simulink model "LCK_old"  (R2018b)
settings: Solver=FixedStepDiscrete  StartTime=0.0  StopTime=inf  FixedStep=0.005  RelTol=1e-3
PostLoadFcn:
  | if any(exist('dsrtsu_mdlpostloadfcn', 'file') ~= 0), dsrtsu_mdlpostloadfcn('Execute', bdroot); end
values from neighbouring files (symbols this model uses):
  C_DEG2RAD = 0.0175    [LCK_Macro.sldd]
  C_KPH2MPS = 0.2778    [LCK_Macro.sldd]
  C_NEARZERO = 0.0001    [LCK_Macro.sldd]
  C_ONE = 1.0    [LCK_Macro.sldd]
  C_RAD2DEG = 57.2958    [LCK_Macro.sldd]
  C_ZERO = 0.0    [LCK_Macro.sldd]
  k_accel_pedal_pos_per_speed_x : value not decoded    [LCK_LogicPara.sldd]
  k_accel_pedal_pos_per_speed_z : value not decoded    [LCK_LogicPara.sldd]
  k_brake_suprress_hold = 1000.0    [LCK_LogicPara.sldd]
  k_driver_appl_torque_filt = 50.0    [LCK_LogicPara.sldd]
  k_driver_suppression_hold_time = 3000.0    [LCK_LogicPara.sldd]
  k_hands_on_wheel_hold_msec = 500.0    [LCK_LogicPara.sldd]
  k_hands_on_wheel_torque_hi = 0.2    [LCK_LogicPara.sldd]
  k_hands_on_wheel_torque_lo = 0.15    [LCK_LogicPara.sldd]
  k_handsoff_delay_cycles = 50.0    [LCK_LogicPara.sldd]
  k_handsoff_torq_Lo_CR = 0.3    [LCK_LogicPara.sldd]
  k_handson_delay_cycles = 5.0    [LCK_LogicPara.sldd]
  k_HighAccel_suppress_hold = 3000.0    [LCK_LogicPara.sldd]
  k_HLR_suprress_hold = 3000.0    [LCK_LogicPara.sldd]
  k_hs_StrAng_CR_threshold_z : value not decoded    [LCK_LogicPara.sldd]
  k_LC_Exit_Switch = 0.0    [LCK_LogicPara.sldd]
  k_LCG_Configured = 1.0    [LCK_LogicPara.sldd]
  k_LCK_A0_Rdy2Act_UseConst = 0.0    [LCK_LogicPara.sldd]
  k_LCK_A0Fac_ActSta : value not decoded    [LCK_CtrlPara.sldd]
  k_LCK_A0Fac_DrvStm : value not decoded    [LCK_CtrlPara.sldd]
  k_LCK_A0Shift_LftCurv : value not decoded    [LCK_CtrlPara.sldd]
  k_LCK_A0Shift_RgtCurv : value not decoded    [LCK_CtrlPara.sldd]
  k_LCK_A0Shift_StraLan = 0.0    [LCK_CtrlPara.sldd]
  k_LCK_A0ShiftFac_Dy_LftCurv : value not decoded    [LCK_CtrlPara.sldd]
  k_LCK_A0ShiftFac_Dy_RgtCurv : value not decoded    [LCK_CtrlPara.sldd]
  k_LCK_A0ShiftFac_Vspd : value not decoded    [LCK_CtrlPara.sldd]
  k_LCK_accel_inhibit_thold = 35.0    [LCK_LogicPara.sldd]
  k_LCK_Active2Ready_Mask = 255.0    [LCK_LogicPara.sldd]
  k_LCK_CvatRateBks : value not decoded    [LCK_CtrlPara.sldd]
  k_LCK_CvatrBks : value not decoded    [LCK_CtrlPara.sldd]
  k_LCK_DFac_Dy : value not decoded    [LCK_CtrlPara.sldd]
  k_LCK_DFac_Dy_Curv : value not decoded    [LCK_CtrlPara.sldd]
  k_LCK_DFac_HaCurCen : value not decoded    [LCK_CtrlPara.sldd]
  k_LCK_DFac_HaCurSid : value not decoded    [LCK_CtrlPara.sldd]
  k_LCK_DFac_HadCurCen : value not decoded    [LCK_CtrlPara.sldd]
  k_LCK_DFac_HadCurSid : value not decoded    [LCK_CtrlPara.sldd]
  k_LCK_DFac_HadStrCen : value not decoded    [LCK_CtrlPara.sldd]
  k_LCK_DFac_HadStrSid : value not decoded    [LCK_CtrlPara.sldd]
  k_LCK_DFac_HaStrCen : value not decoded    [LCK_CtrlPara.sldd]
  k_LCK_DFac_HaStrSid : value not decoded    [LCK_CtrlPara.sldd]
  k_LCK_DFac_Rad : value not decoded    [LCK_CtrlPara.sldd]
  k_LCK_DFac_SA_CurCen : value not decoded    [LCK_CtrlPara.sldd]
  k_LCK_DFac_SA_CurSid : value not decoded    [LCK_CtrlPara.sldd]
  k_LCK_DFac_SA_StrCen : value not decoded    [LCK_CtrlPara.sldd]
  k_LCK_DFac_SA_StrSid : value not decoded    [LCK_CtrlPara.sldd]
  k_LCK_DFac_SS_CurCen : value not decoded    [LCK_CtrlPara.sldd]
  k_LCK_DFac_SS_CurSid : value not decoded    [LCK_CtrlPara.sldd]
  k_LCK_DFac_SS_StrCen : value not decoded    [LCK_CtrlPara.sldd]
  k_LCK_DFac_SS_StrSid : value not decoded    [LCK_CtrlPara.sldd]
  k_LCK_DFac_Vspd : value not decoded    [LCK_CtrlPara.sldd]
  k_LCK_DlyTm_DrvStim = 0.2    [LCK_CtrlPara.sldd]
  k_LCK_DTermMax = 2.0    [LCK_CtrlPara.sldd]
  k_LCK_DyBks_Curv : value not decoded    [LCK_CtrlPara.sldd]
  k_LCK_Enable_POOnly = 1.0    [LCK_LogicPara.sldd]
  k_LCK_Entry_DistBuffer = 0.1    [LCK_LogicPara.sldd]
  k_LCK_Fac_Vspd2RngThr_FalRec = 0.23    [LCK_CtrlPara.sldd]
  k_LCK_Ffw_CvatSwh = 0.0    [LCK_CtrlPara.sldd]
  k_LCK_Ffw_DyBks : value not decoded    [LCK_CtrlPara.sldd]
  k_LCK_Ffw_TimCon_CmdFlt = 0.0    [LCK_CtrlPara.sldd]
  k_LCK_FfwDeltaFac_Rad_Lft : value not decoded    [LCK_CtrlPara.sldd]
  k_LCK_FfwDeltaFac_Rad_Rgt : value not decoded    [LCK_CtrlPara.sldd]
  k_LCK_FfwDeltaFac_Vspd : value not decoded    [LCK_CtrlPara.sldd]
  k_LCK_FfwFac_CvatRate_Lft : value not decoded    [LCK_CtrlPara.sldd]
  k_LCK_FfwFac_CvatRate_Rgt : value not decoded    [LCK_CtrlPara.sldd]
  k_LCK_FfwFac_Dy : value not decoded    [LCK_CtrlPara.sldd]
  k_LCK_FfwFac_Rad_Lft : value not decoded    [LCK_CtrlPara.sldd]
  k_LCK_FfwFac_Rad_Rgt : value not decoded    [LCK_CtrlPara.sldd]
  k_LCK_FfwFac_Vspd : value not decoded    [LCK_CtrlPara.sldd]
  k_LCK_FfwTorq_Cvat : value not decoded    [LCK_CtrlPara.sldd]
  k_LCK_HAFac_ActSta : value not decoded    [LCK_CtrlPara.sldd]
  k_LCK_HAFac_DrvStm : value not decoded    [LCK_CtrlPara.sldd]
  k_LCK_HaloTime = 2000.0    [LCK_LogicPara.sldd]
  k_LCK_HaloTime_Switch = 0.0    [LCK_LogicPara.sldd]
  k_LCK_HARFac_ActSta : value not decoded    [LCK_CtrlPara.sldd]
  k_LCK_HARFac_DrvStm : value not decoded    [LCK_CtrlPara.sldd]
  k_LCK_Hed_DyBks : value not decoded    [LCK_CtrlPara.sldd]
  k_LCK_HedAngDiffX : value not decoded    [LCK_CtrlPara.sldd]
  k_LCK_HedAngRateDiffX : value not decoded    [LCK_CtrlPara.sldd]
  k_LCK_HndsOnWhel_DlyTm_Idl2Rdy = 0.0    [LCK_LogicPara.sldd]
  k_LCK_host_veh_width = 1.86    [LCK_LogicPara.sldd]
  k_LCK_Idle2Ready_Mask = 239.0    [LCK_LogicPara.sldd]
  k_LCK_Junc_SusTime = 1.0    [LCK_LogicPara.sldd]
  k_LCK_KpKdDecSlopeLmt = 10.0    [LCK_CtrlPara.sldd]
  k_LCK_KpKdIncSlopeLmt = 5.0    [LCK_CtrlPara.sldd]
  k_LCK_Lat_Ctrl_DFac_Lft = 1.0    [LCK_CtrlPara.sldd]
  k_LCK_Lat_Ctrl_DFac_Rgt = 1.05    [LCK_CtrlPara.sldd]
  k_LCK_Lat_Ctrl_Kd = 0.8    [LCK_CtrlPara.sldd]
  k_LCK_Lat_Ctrl_Ki = 0.5    [LCK_CtrlPara.sldd]
  k_LCK_Lat_Ctrl_Kp = 0.7    [LCK_CtrlPara.sldd]
  k_LCK_Lat_Ctrl_Kp_NearGain = 0.7    [LCK_CtrlPara.sldd]
  k_LCK_Lat_Ctrl_PFac_Lft = 1.0    [LCK_CtrlPara.sldd]
  k_LCK_Lat_Ctrl_PFac_Rgt = 1.05    [LCK_CtrlPara.sldd]
  k_LCK_Lat_Ctrl_TimCon_CmdFlt = 5.0    [LCK_CtrlPara.sldd]
  k_LCK_Lat_DFac_Rad : value not decoded    [LCK_CtrlPara.sldd]
  k_LCK_Lat_DFac_SS_Cur : value not decoded    [LCK_CtrlPara.sldd]
  k_LCK_Lat_DFac_SS_Str : value not decoded    [LCK_CtrlPara.sldd]
  k_LCK_Lat_DFac_Vspd : value not decoded    [LCK_CtrlPara.sldd]
  k_LCK_Lat_DyBks : value not decoded    [LCK_CtrlPara.sldd]
  k_LCK_Lat_IFac_Rad : value not decoded    [LCK_CtrlPara.sldd]
  k_LCK_Lat_IFac_Vspd : value not decoded    [LCK_CtrlPara.sldd]
  k_LCK_Lat_ILmtFac_Dy_CurvLan : value not decoded    [LCK_CtrlPara.sldd]
  k_LCK_Lat_ILmtFac_Dy_StraLan : value not decoded    [LCK_CtrlPara.sldd]
  k_LCK_Lat_ILmtFac_Rad : value not decoded    [LCK_CtrlPara.sldd]
  k_LCK_Lat_ILmtFac_Rad_NearGain = 1.0    [LCK_CtrlPara.sldd]
  k_LCK_Lat_ILmtFac_Vspd_CurvLan : value not decoded    [LCK_CtrlPara.sldd]
  k_LCK_Lat_ILmtFac_Vspd_StraLan : value not decoded    [LCK_CtrlPara.sldd]
  k_LCK_Lat_ITermLmt_Dy = 1.0    [LCK_CtrlPara.sldd]
  k_LCK_Lat_KpKdDecSlopeLmt = 10.0    [LCK_CtrlPara.sldd]
  k_LCK_Lat_KpKdIncSlopeLmt = 10.0    [LCK_CtrlPara.sldd]
  k_LCK_Lat_PFac_Dy_InnLftCur : value not decoded    [LCK_CtrlPara.sldd]
  k_LCK_Lat_PFac_Dy_InnRgtCur : value not decoded    [LCK_CtrlPara.sldd]
  k_LCK_Lat_PFac_Dy_OutLftCur : value not decoded    [LCK_CtrlPara.sldd]
  k_LCK_Lat_PFac_Dy_OutRgtCur : value not decoded    [LCK_CtrlPara.sldd]
  k_LCK_Lat_PFac_Dy_Str : value not decoded    [LCK_CtrlPara.sldd]
  k_LCK_Lat_PFac_Rad : value not decoded    [LCK_CtrlPara.sldd]
  ... (+158 more)
undefined symbols (not defined in the file or in its folder): k_LCK_CurvBks, K_LCK_SPA0A1A2_LMRngCmp_y
libraries: LateralControl_fcns_lib x58, simulink x22
(part 32 of 45)

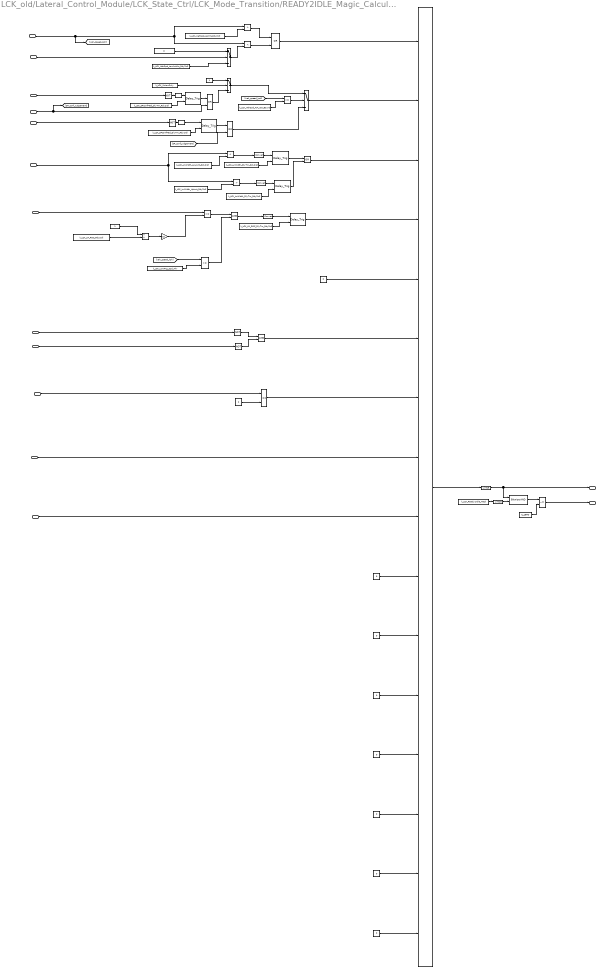
== system LCK_old/Lateral_Control_Module/LCK_State_Ctrl/LCK_Mode_Transition/READY2IDLE_Magic_Calculation ==
  note: LKATrqOvrlTrqDStat
      | 0: inactive
      | 1: active
      | 2:Temporary inhibit
      | 3:Permanantly failed
  veh_speed_kph : Inport
  TJA_Switch : Inport  Port=2
  SP_valid_low_spd : Inport  Port=3
  SP_valid_high_spd : Inport  Port=4
  SP_conf_Judgement : Inport  Port=5
  curr_lane_width : Inport  Port=6
  SPP_A2 : Inport  Port=7
  LCK_Feature_Enabled : Inport  Port=8
  ERROR_CONDITION : Inport  Port=9
  LKATrqOvrlTrqDStat : Inport  Port=10
  YawRate_Over_Threshold : Inport  Port=11
  Short_LM_Range : Inport  Port=12
  Constant{1..3,18} (4 alike) : Constant  Tag={'output',{'type','Int32'},'date',737237.63745989581}  Description=_GWMAB30P3.LCK.000_24_  Value=0
  Constant10 : Constant  Tag={'output',{'class','ESR_VC/CONST','type','UInt16'},'date',737194.71866488422}  Description=_GWMAB30P2.LCK.000_1067_  Value=0
  Constant22 : Constant  Tag={'output',{'type','Int32'},'date',737184.60397321754}  Description=_GWMAB30P2.LCK.000_1073_
  Constant24 : Constant  Tag={'output',{'type','Int32'},'date',737237.63746031246}  Description=_GWMAB30P3.LCK.000_25_  Value=0
  Constant29 : Constant  Tag={'output',{'type','Int32'},'date',737237.63746063656}  Description=_GWMAB30P3.LCK.000_26_  Value=0
  Constant4 : Constant  Tag={'output',{'type','Int32'},'date',737296.81489093753}  Description=_GWMAB30P2.LCK.000_1072_
  Constant55 : Constant  Tag={'output',{'type','Int32'},'date',737292.69766020833}  Description=_GWMAB30P4.LCK.000_120_  Value=2
  Constant8 : Constant  Tag={'output',{'class','ESR_VC/CONST','type','UInt16'},'date',737194.71861182875}  Description=_GWMAB30P2.LCK.000_1084_  Value=0
  Data Type Conversion13 : DataTypeConversion  Description=_GWMAB30P4.LCK.000_124_  OutDataTypeStr=uint16
  Data Type Conversion15 : DataTypeConversion  Description=_GWMAB30P4.LCK.000_126_
  Data Type Conversion22 : DataTypeConversion  Description=_GWMAB30P4.LCK.000_133_
  Data Type Conversion31 : DataTypeConversion  Description=_GWMAB30P4.LCK.000_143_
  Data Type Conversion6 : DataTypeConversion  Description=_GWMAB30P4.LCK.000_148_
  Data Type Conversion7 : DataTypeConversion  Description=_GWMAB30P4.LCK.000_149_
  Data Type Conversion90 : DataTypeConversion  OutDataTypeStr=uint16
  Delay_Trig{,1..4} (5 alike) : LateralControl_fcns_lib/Delay_Trig  SystemSampleTime=-1
  Divide : Product  Inputs=*/
  Gain : Gain  Gain=0.5
  IDLE2READY_Magic : LateralControl_fcns_lib/Bit_To_Integer_16  SystemSampleTime=-1
  Logical Operator1 : Logic  Tag={'date',737184.60397571756}  Description=_GWMAB30P2.LCK.000_1091_  Operator=NOT  Inputs=1  AllPortsSameDT=off  OutDataTypeStr=boolean
  Logical Operator17 : Logic  Tag={'date',737237.63746609958}  Description=_GWMAB30P3.LCK.000_60_  Operator=NOT  Inputs=1  AllPortsSameDT=off  OutDataTypeStr=boolean
  Logical Operator20 : Logic  Tag={'date',737184.60397694446}  Description=_GWMAB30P2.LCK.000_1101_  Operator=OR  AllPortsSameDT=off  OutDataTypeStr=boolean
  Logical Operator22 : Logic  AllPortsSameDT=off  OutDataTypeStr=boolean
  Logical Operator27 : Logic  Tag={'date',737237.63746688655}  Description=_GWMAB30P3.LCK.000_64_  Operator=OR  AllPortsSameDT=off  OutDataTypeStr=boolean
  Logical Operator45 : Logic  Tag={'date',737184.60398017359}  Description=_GWMAB30P2.LCK.000_1127_  Operator=OR  AllPortsSameDT=off  OutDataTypeStr=boolean
  Logical Operator46 : Logic  Tag={'date',737184.60398031247}  Description=_GWMAB30P2.LCK.000_1128_  Operator=NOT  Inputs=1  AllPortsSameDT=off  OutDataTypeStr=boolean
  Logical Operator47 : Logic  Tag={'date',737184.60398042819}  Description=_GWMAB30P2.LCK.000_1129_  AllPortsSameDT=off  OutDataTypeStr=boolean
  Logical Operator55 : Logic  Tag={'date',737237.63746870367}  Description=_GWMAB30P3.LCK.000_73_  Operator=OR  AllPortsSameDT=off  OutDataTypeStr=boolean
  Logical Operator56 : Logic  Tag={'date',737237.63746884256}  Description=_GWMAB30P3.LCK.000_74_  Operator=NOT  Inputs=1  AllPortsSameDT=off  OutDataTypeStr=boolean
  Ready2IdleBitwise Operator1 : simulink/Logic and Bit Operations/Bitwise Operator  logicop=AND  UseBitMask=off  NumInputPorts=2  BitMask=k_LCK_Ready2Idle_Mask  BitMaskRealWorld=Stored Integer
  Relational Operator1 : RelationalOperator  OutDataTypeStr=boolean  RndMeth=Nearest
  Relational Operator14 : RelationalOperator  Tag={'date',737184.60398192133}  Description=_GWMAB30P2.LCK.000_1141_  Operator=>  OutDataTypeStr=boolean  RndMeth=Nearest
  Relational Operator18 : RelationalOperator  Tag={'date',737184.60398240737}  Description=_GWMAB30P2.LCK.000_1145_  Operator=<  OutDataTypeStr=boolean  RndMeth=Nearest
  Relational Operator20 : RelationalOperator  Tag={'date',737184.6039827778}  Description=_GWMAB30P2.LCK.000_1148_  Operator=<  OutDataTypeStr=boolean  RndMeth=Nearest
  Relational Operator21 : RelationalOperator  Tag={'date',737184.60398289352}  Description=_GWMAB30P2.LCK.000_1149_  Operator=>  OutDataTypeStr=boolean  RndMeth=Nearest
  Relational Operator22 : RelationalOperator  Tag={'date',737184.60398302088}  Description=_GWMAB30P2.LCK.000_1150_  OutDataTypeStr=boolean  RndMeth=Nearest
  Relational Operator27 : RelationalOperator  Tag={'date',737292.6976654398}  Description=_GWMAB30P4.LCK.000_183_  Operator===  OutDataTypeStr=boolean  RndMeth=Nearest
  Relational Operator7 : RelationalOperator  Tag={'date',737184.6039870833}  Description=_GWMAB30P2.LCK.000_1183_  Operator=<=  OutDataTypeStr=boolean  RndMeth=Nearest
  Relational_Operator1 : RelationalOperator  Tag={'date',737184.60398746526}  Description=_GWMAB30P2.LCK.000_1186_  Operator=~=  OutDataTypeStr=boolean  RndMeth=Nearest
  Switch11 : Switch  Tag={'output',{'type','UInt16'},'threshold',{'type','Int32'},'date',737243.53932971065}  Description=_GWMAB30P3.LCK.000_112_  Threshold=0.5
  Switch4 : Switch  Tag={'output',{'type','Bool'},'threshold',{'type','Int32','scalar',1},'date',737395.45390497684}  Description=_GWMAB30P2.LCK.000_1194_  Threshold=0.5
  Switch8 : Switch  Tag={'output',{'inheritscaling',1},'threshold',{'type','Int32','scalar',1},'date',737189.77895010414}  Description=_GWMAB30P2.LCK.000_1198_  Threshold=0.5
  ZERO1 : Constant  Tag={'output',{'name','$P','class','EXTERN_CONST','type','Bool'},'date',737395.73574942129}  Description=_GWMAB30P2.LCK.000_1206_  Value=C_ZERO  SampleTime=-1
  k_LCK_LM_ROC_DlyTm_Rdy2Idl : Constant  Tag={'output',{'name','$P','class','EXTERN_CAL','type','UInt8'},'date',737246.86453901615}  Description=_GWMAB30P2.LCK.000_1238_  Value=k_LCK_LM_ROC_DlyTm_Rdy2Idl
  k_LCK_LM_ROC_Rdy2Idl : Constant  Tag={'output',{'name','$P','class','EXTERN_CAL','type','UInt16'},'date',737246.86453862267}  Description=_GWMAB30P2.LCK.000_1240_  Value=k_LCK_LM_ROC_Rdy2Idl
  k_LCK_LnWidth_DlyTm_Rdy2Idl : Constant  Tag={'output',{'name','$P','class','EXTERN_CAL','type','UInt8'},'date',737246.86453621532}  Description=_GWMAB30P2.LCK.000_1245_  Value=k_LCK_LnWidth_DlyTm_Rdy2Idl
  k_LCK_LnWidth_DlyTm_Rdy2Idl1 : Constant  Tag={'output',{'name','$P','class','EXTERN_CAL','type','UInt8'},'date',737246.86453643523}  Description=_GWMAB30P2.LCK.000_1246_  Value=k_LCK_LnWidth_DlyTm_Rdy2Idl
  k_LCK_LnWidth_LowLmt_Rdy2Idl : Constant  Tag={'output',{'name','$P','class','EXTERN_CAL','type','Float32'},'date',737246.86453582172}  Description=_GWMAB30P2.LCK.000_1248_  Value=k_LCK_LnWidth_LowLmt_Rdy2Idl
  k_LCK_LnWidth_UpLmt_Rdy2Idl : Constant  Tag={'output',{'name','$P','class','EXTERN_CAL','type','Float32'},'date',737246.86453543976}  Description=_GWMAB30P2.LCK.000_1250_  Value=k_LCK_LnWidth_UpLmt_Rdy2Idl
  k_LCK_LowRng_Spd_Thr1 : Constant  Value=k_LCK_LowRng_Spd_Thr
  k_LCK_Ready2Idle_Mask : Constant  Value=k_LCK_Ready2Idle_Mask
  k_LCK_SPconfMed_DlyTm_Rdy2Idl1 : Constant  Tag={'output',{'name','$P','class','EXTERN_CAL','type','Float32'},'date',737531.64186515042}  Description=_GWMAB30P3.LCK.000_146_  Value=k_LCK_SPconfMed_DlyTm_Rdy2Idl
  k_LCK_SPconfMed_DlyTm_Rdy2Idl2 : Constant  Tag={'output',{'name','$P','class','EXTERN_CAL','type','Float32'},'date',737531.64211655094}  Description=_GWMAB30P3.LCK.000_147_  Value=k_LCK_SPconfMed_DlyTm_Rdy2Idl
  k_LCK_VehSpd_LowLmtFus_Rdy2Idl : Constant  Tag={'output',{'type','Int32'},'date',737237.63748364581}  Description=_GWMAB30P3.LCK.000_149_  Value=0
  k_LCK_VehSpd_LowlmtVis_Rdy2Idl : Constant  Tag={'output',{'name','$P','class','EXTERN_CAL','type','UInt16'},'date',737246.86429206014}  Description=_GWMAB30P3.LCK.000_151_  Value=k_LCK_VehSpd_LowlmtVis_Rdy2Idl
  k_LCK_VehSpd_TJA_ICA_Bound1 : Constant  Tag={'output',{'name','$P','class','EXTERN_CAL','type','UInt16'},'date',737246.86429164349}  Description=_GWMAB30P2.LCK.000_1265_  Value=k_LCK_VehSpd_TJA_ICA_Bound
  k_LCK_VehSpd_Uplmt_Rdy2Idl : Constant  Tag={'output',{'name','$P','class','EXTERN_CAL','type','UInt16'},'date',737246.86429093755}  Description=_GWMAB30P2.LCK.000_1267_  Value=k_LCK_VehSpd_Uplmt_Rdy2Idl
  k_LCK_VisionOnly : Constant  Tag={'output',{'name','$P','class','EXTERN_CAL','type','Bool'},'date',737246.86429052078}  Description=_GWMAB30P2.LCK.000_1268_  Value=k_LCK_VisionOnly
  READY2IDLE_Magic_Out : Outport
  READY2IDLE : Outport  Port=2
  wires:
  Logical Operator20/1 -> IDLE2READY_Magic/3
  Constant24/1 -> IDLE2READY_Magic/13
  Logical Operator46/1 -> Logical Operator47/2
  Delay_Trig4/1 -> IDLE2READY_Magic/4
  k_LCK_VehSpd_LowLmtFus_Rdy2Idl/1 -> Switch11/1
  Delay_Trig/1 -> Logical Operator27/1
  Data Type Conversion13/1 -> READY2IDLE_Magic_Out/1, Ready2IdleBitwise Operator1/1
  k_LCK_VehSpd_LowlmtVis_Rdy2Idl/1 -> Switch11/3
  Constant1/1 -> IDLE2READY_Magic/10
  k_LCK_Ready2Idle_Mask/1 -> Data Type Conversion90/1
  Logical Operator56/1 -> Data Type Conversion31/1
  Switch4/1 -> IDLE2READY_Magic/2
  veh_speed_kph/1 -> [veh_speed_kph], Relational Operator14/1, Relational Operator18/1
  Data Type Conversion15/1 -> Delay_Trig1/1
  Data Type Conversion31/1 -> Delay_Trig/1
  curr_lane_width/1 -> Relational Operator21/1, Relational Operator20/1
  Logical Operator55/1 -> Switch4/3
  Data Type Conversion7/1 -> Delay_Trig4/1
  Constant29/1 -> IDLE2READY_Magic/16
  k_LCK_SPconfMed_DlyTm_Rdy2Idl1/1 -> Delay_Trig1/2
  Relational Operator14/1 -> Logical Operator45/1
  k_LCK_LM_ROC_DlyTm_Rdy2Idl/1 -> Delay_Trig4/2
  Logical Operator47/1 -> IDLE2READY_Magic/6
  Ready2IdleBitwise Operator1/1 -> Relational_Operator1/1
  [SP_conf_Judgement] -> Logical Operator55/2
  Logical Operator17/1 -> Data Type Conversion15/1
  YawRate_Over_Threshold/1 -> IDLE2READY_Magic/8
  Relational Operator1/1 -> Logical Operator22/2
  Delay_Trig2/1 -> Logical Operator20/1
  Constant3/1 -> IDLE2READY_Magic/5
  Delay_Trig1/1 -> Logical Operator55/1
  Relational Operator21/1 -> Data Type Conversion22/1
  k_LCK_SPconfMed_DlyTm_Rdy2Idl2/1 -> Delay_Trig/2
  Constant18/1 -> IDLE2READY_Magic/12
  Switch8/1 -> Switch4/1
  Relational Operator18/1 -> Logical Operator45/2
  Constant10/1 -> IDLE2READY_Magic/15
  Switch11/1 -> Relational Operator18/2
  k_LCK_LnWidth_LowLmt_Rdy2Idl/1 -> Relational Operator20/2
  Constant22/1 -> Switch8/1
  Logical Operator45/1 -> IDLE2READY_Magic/1
  Delay_Trig3/1 -> Logical Operator20/2
  k_LCK_LnWidth_DlyTm_Rdy2Idl/1 -> Delay_Trig2/2
  ZERO1/1 -> Relational_Operator1/2
  k_LCK_LnWidth_DlyTm_Rdy2Idl1/1 -> Delay_Trig3/2
  Data Type Conversion6/1 -> Delay_Trig2/1
  k_LCK_VehSpd_Uplmt_Rdy2Idl/1 -> Relational Operator14/2
  k_LCK_LnWidth_UpLmt_Rdy2Idl/1 -> Relational Operator21/2
  Relational Operator20/1 -> Data Type Conversion6/1
  Logical Operator22/1 -> Data Type Conversion7/1
  [veh_speed_kph] -> Relational Operator7/1
  Relational Operator22/1 -> Logical Operator22/1
  Logical Operator1/1 -> Logical Operator47/1
  Data Type Conversion22/1 -> Delay_Trig3/1
  Relational Operator7/1 -> Switch4/2
  Logical Operator27/1 -> Switch8/3
  k_LCK_VehSpd_TJA_ICA_Bound1/1 -> Relational Operator7/2
  Data Type Conversion90/1 -> Ready2IdleBitwise Operator1/2
  IDLE2READY_Magic/1 -> Data Type Conversion13/1
  Constant8/1 -> IDLE2READY_Magic/14
  SP_valid_low_spd/1 -> Logical Operator56/1
  SP_conf_Judgement/1 -> [SP_conf_Judgement], Logical Operator27/2
  SPP_A2/1 -> Relational Operator22/1
  SP_valid_high_spd/1 -> Logical Operator17/1
  Relational_Operator1/1 -> READY2IDLE/1
  TJA_Switch/1 -> Switch11/2
  k_LCK_VisionOnly/1 -> Switch8/2
  Relational Operator27/1 -> IDLE2READY_Magic/7
  ERROR_CONDITION/1 -> Logical Operator46/1
  LCK_Feature_Enabled/1 -> Logical Operator1/1
  k_LCK_LowRng_Spd_Thr1/1 -> Relational Operator1/2
  [veh_speed_kph] -> Relational Operator1/1
  LKATrqOvrlTrqDStat/1 -> Relational Operator27/1
  Constant55/1 -> Relational Operator27/2
  Short_LM_Range/1 -> IDLE2READY_Magic/9
  Constant2/1 -> IDLE2READY_Magic/11
  Divide/1 -> Gain/1
  Constant4/1 -> Divide/1
  Gain/1 -> Relational Operator22/2
  k_LCK_LM_ROC_Rdy2Idl/1 -> Divide/2
